simulink model "gm_uz_pmsm_model_9ph_vnl"  (R2021b)
settings: Solver=FixedStepAuto  StartTime=0.0  StopTime=0.8  RelTol=1e-3
PreLoadFcn:
  | uz_pmsm_model_9ph_init_parameter
undefined symbols (not defined in the file or in its folder): a, b, c, friction_coefficient, inertia, k_i_d, k_i_q, k_p_d, k_p_q, Kpd, L_d, L_o1, L_o2, L_q, L_x1, L_x2, L_y1, L_y2, L_zero, polepair, psi_pm, R_1, static_friction_torque, Tnd, ts
libraries: hdlmdlgenlib x191, hdlsllib x90, dspsigops x19, simulink x17, slpidlib x2, spsAlphaBetaZerotodq0Lib x1, pid_lib x1, spsdq0toAlphaBetaZeroLib x1
(part 1 of 7)
settings Model: Creator=ts  LastModifiedBy=valen
settings SolverCC: AlgebraicLoopSolver=TrustRegion  AutoInsertRateTranBlk=on
settings DataIOCC: LimitDataPoints=on  SaveOutput=off  SaveTime=off
settings OptimizationCC: BlockReduction=off  ConditionallyExecuteInputs=off  DefaultParameterBehavior=Inlined  LifeSpan=inf
settings DebuggingCC: AlgebraicLoopMsg=error  ArtificialAlgebraicLoopMsg=none  InheritedTsInSrcMsg=none  SingleTaskRateTransMsg=error  AllowSymbolicDim=off  StrictBusMsg=ErrorOnBusTreatedAsVector  SFUnexpectedBacktrackingDiag=warning  SFNoUnconditionalDefaultTransitionDiag=warning  SFExecutionAtInitializationDiag=none  SFMachineParentedDataDiag=warning  ArithmeticOperatorsInVariantConditions=warning
settings HardwareCC: ProdBitPerPointer=32  ProdBitPerSizeT=32  ProdBitPerPtrDiffT=32  ProdLargestAtomicFloat=None  ProdIntDivRoundTo=Undefined  ProdEndianess=Unspecified  ProdWordSize=32  ProdHWDeviceType=ASIC/FPGA->ASIC/FPGA  ProdEqTarget=off
settings SFSimCC: SimUseLocalCustomCode=off  CustomCodeUndefinedFunction=UseInterfaceOnly
settings RTWCC: RTWUseLocalCustomCode=off
settings CodeAppCC: StateflowObjectComments=on
settings GRTTargetCC: TargetLangStandard=C89/C90 (ANSI)
settings ConfigComp: CovScope=ReferencedModels  CovMetricSettings=dw  CovSaveCumulativeToWorkspaceVar=on  CovSaveSingleToWorkspaceVar=on  CovExternalEMLEnable=off  CovSFcnEnable=off

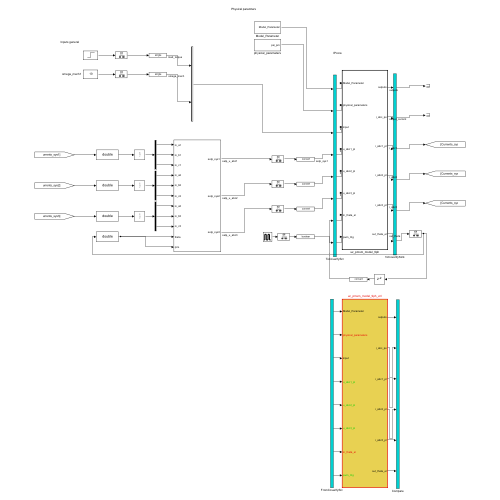
[thumbnail: Simulink's stored preview of the top-level diagram]
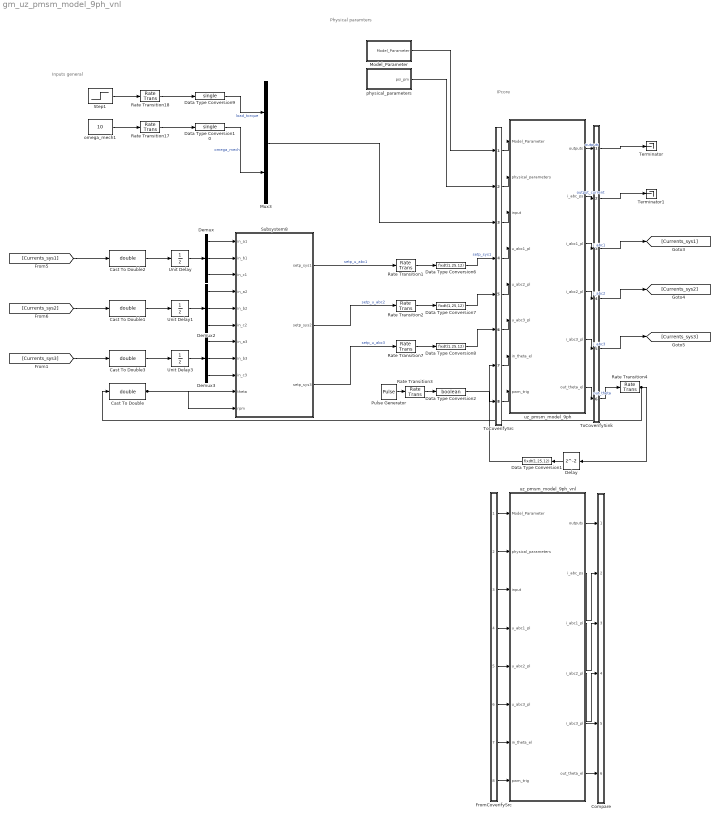
== system gm_uz_pmsm_model_9ph_vnl ==
  note: IPcore
  note: Physical paramters
  note: Inputs general
  Cast To Double{,1..3} (4 alike) : DataTypeConversion  OutDataTypeStr=double
  Compare : Subsystem
      mask Display: disp('')
  Data Type Conversion{1,6..8} (4 alike) : DataTypeConversion  OutDataTypeStr=fixdt(1,25,12)  RndMeth=Nearest
  Data Type Conversion10 : DataTypeConversion  OutDataTypeStr=single  RndMeth=Nearest
  Data Type Conversion2 : DataTypeConversion  OutDataTypeStr=boolean  RndMeth=Nearest
  Data Type Conversion9 : DataTypeConversion  OutDataTypeStr=single  RndMeth=Nearest
  Delay : Delay
  Demux : Demux  Outputs=3
  Demux2 : Demux  Outputs=3
  Demux3 : Demux  Outputs=3
  FromCoverifySrc : Subsystem
      mask Display: disp('')
  Model_Parameter : Subsystem
  Mux3 : Mux  Inputs=2
  Pulse Generator : DiscretePulseGenerator  PulseType=Time based  Period=1e-9  PulseWidth=50
  Rate Transition{1..4,7,17..18} (7 alike) : RateTransition  OutPortSampleTime=ts
  Step1 : Step  Time=0.25  After=20  SampleTime=0
  Subsystem8 : Subsystem
  Terminator : Terminator
  Terminator1 : Terminator
  ToCoverifySink : Subsystem
      mask Display: disp('')
  ToCoverifySrc : Subsystem
      mask Display: disp('')
  Unit Delay : UnitDelay  SampleTime=-1  HasFrameUpgradeWarning=on
  Unit Delay1 : UnitDelay  SampleTime=-1  HasFrameUpgradeWarning=on
  Unit Delay3 : UnitDelay  SampleTime=-1  HasFrameUpgradeWarning=on
  omega_mech1 : Constant  Value=10
  physical_parameters : Subsystem
  uz_pmsm_model_9ph : Subsystem  TreatAsAtomicUnit=on
  uz_pmsm_model_9ph_vnl : Subsystem  TreatAsAtomicUnit=on
  wires:
  omega_mech1/1 -> Rate Transition17/1
  Rate Transition18/1 -> Data Type Conversion9/1
  Step1/1 -> Rate Transition18/1
  Data Type Conversion10/1 -> Mux3/2  "omega_mech"
  Rate Transition17/1 -> Data Type Conversion10/1
  Data Type Conversion9/1 -> Mux3/1  "load_torque"
  Delay/1 -> Data Type Conversion1/1
  Subsystem8/1(setp_sys1) -> Rate Transition1/1  "setp_u_abc1"
  Subsystem8/2(setp_sys2) -> Rate Transition2/1  "setp_u_abc2"
  Subsystem8/3(setp_sys3) -> Rate Transition7/1  "setp_u_abc3"
  Unit Delay3/1 -> Demux3/1
  Demux/2 -> Subsystem8/2(in_b1)
  Demux2/1 -> Subsystem8/4(in_a2)
  Demux3/2 -> Subsystem8/8(in_b3)
  Unit Delay1/1 -> Demux2/1
  Demux/3 -> Subsystem8/3(in_c1)
  [Currents_sys1] -> Cast To Double2/1
  [Currents_sys2] -> Cast To Double1/1
  Demux3/3 -> Subsystem8/9(in_c3)
  Unit Delay/1 -> Demux/1
  [Currents_sys3] -> Cast To Double3/1
  Demux3/1 -> Subsystem8/7(in_a3)
  Demux/1 -> Subsystem8/1(in_a1)
  Demux2/2 -> Subsystem8/5(in_b2)
  Demux2/3 -> Subsystem8/6(in_c2)
  Cast To Double/1 -> Subsystem8/11(rpm), Subsystem8/10(theta)
  Cast To Double1/1 -> Unit Delay1/1
  Cast To Double2/1 -> Unit Delay/1
  Cast To Double3/1 -> Unit Delay3/1
  Rate Transition1/1 -> Data Type Conversion6/1
  Rate Transition2/1 -> Data Type Conversion7/1
  Rate Transition7/1 -> Data Type Conversion8/1
  Rate Transition3/1 -> Data Type Conversion2/1
  Pulse Generator/1 -> Rate Transition3/1
  Rate Transition4/1 -> Delay/1, Cast To Double/1
  ToCoverifySrc/1(out1) -> uz_pmsm_model_9ph/1(Model_Parameter)
  ToCoverifySrc/2(out2) -> uz_pmsm_model_9ph/2(physical_parameters)
  ToCoverifySrc/3(out3) -> uz_pmsm_model_9ph/3(input)
  ToCoverifySrc/4(out4) -> uz_pmsm_model_9ph/4(u_abc1_pl)
  ToCoverifySrc/5(out5) -> uz_pmsm_model_9ph/5(u_abc2_pl)
  ToCoverifySrc/6(out6) -> uz_pmsm_model_9ph/6(u_abc3_pl)
  ToCoverifySrc/7(out7) -> uz_pmsm_model_9ph/7(in_theta_el)
  ToCoverifySrc/8(out8) -> uz_pmsm_model_9ph/8(pwm_trig)
  uz_pmsm_model_9ph/1(outputs) -> ToCoverifySink/1(in1)  "outputs"
  uz_pmsm_model_9ph/2(i_abc_ps) -> ToCoverifySink/2(in2)  "output_current"
  uz_pmsm_model_9ph/3(i_abc1_pl) -> ToCoverifySink/3(in3)  "i_abc1"
  uz_pmsm_model_9ph/4(i_abc2_pl) -> ToCoverifySink/4(in4)  "i_abc2"
  uz_pmsm_model_9ph/5(i_abc3_pl) -> ToCoverifySink/5(in5)  "i_abc3"
  uz_pmsm_model_9ph/6(out_theta_el) -> ToCoverifySink/6(in6)  "out_theta"
  Model_Parameter/1(Model_Parameter) -> ToCoverifySrc/1(in1)
  physical_parameters/1(psi_pm) -> ToCoverifySrc/2(in2)
  Mux3/1 -> ToCoverifySrc/3(in3)
  Data Type Conversion6/1 -> ToCoverifySrc/4(in4)  "setp_sys1"
  Data Type Conversion7/1 -> ToCoverifySrc/5(in5)
  Data Type Conversion8/1 -> ToCoverifySrc/6(in6)
  Data Type Conversion1/1 -> ToCoverifySrc/7(in7)
  Data Type Conversion2/1 -> ToCoverifySrc/8(in8)
  ToCoverifySink/1(out1) -> Terminator/1
  ToCoverifySink/2(out2) -> Terminator1/1
  ToCoverifySink/3(out3) -> [Currents_sys1]
  ToCoverifySink/4(out4) -> [Currents_sys2]
  ToCoverifySink/5(out5) -> [Currents_sys3]
  ToCoverifySink/6(out6) -> Rate Transition4/1
  FromCoverifySrc/1(out1) -> uz_pmsm_model_9ph_vnl/1(Model_Parameter)
  FromCoverifySrc/2(out2) -> uz_pmsm_model_9ph_vnl/2(physical_parameters)
  FromCoverifySrc/3(out3) -> uz_pmsm_model_9ph_vnl/3(input)
  FromCoverifySrc/4(out4) -> uz_pmsm_model_9ph_vnl/4(u_abc1_pl)
  FromCoverifySrc/5(out5) -> uz_pmsm_model_9ph_vnl/5(u_abc2_pl)
  FromCoverifySrc/6(out6) -> uz_pmsm_model_9ph_vnl/6(u_abc3_pl)
  FromCoverifySrc/7(out7) -> uz_pmsm_model_9ph_vnl/7(in_theta_el)
  FromCoverifySrc/8(out8) -> uz_pmsm_model_9ph_vnl/8(pwm_trig)
  uz_pmsm_model_9ph_vnl/1(outputs) -> Compare/1(in1)
  uz_pmsm_model_9ph_vnl/2(i_abc_ps) -> Compare/2(in2)
  uz_pmsm_model_9ph_vnl/3(i_abc1_pl) -> Compare/3(in3)
  uz_pmsm_model_9ph_vnl/4(i_abc2_pl) -> Compare/4(in4)
  uz_pmsm_model_9ph_vnl/5(i_abc3_pl) -> Compare/5(in5)
  uz_pmsm_model_9ph_vnl/6(out_theta_el) -> Compare/6(in6)

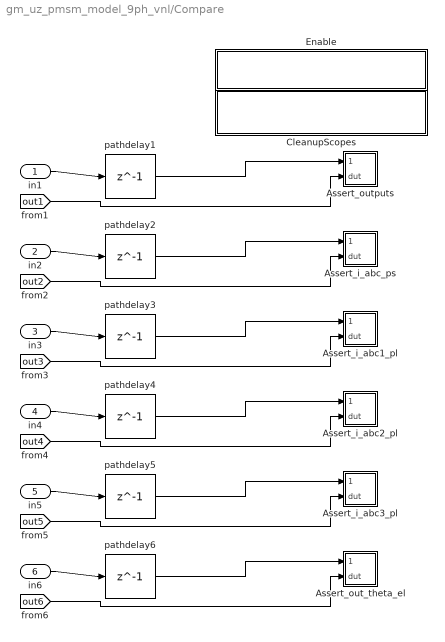
== system gm_uz_pmsm_model_9ph_vnl/Compare ==
  in1 : Inport
  in2 : Inport  Port=2
  in3 : Inport  Port=3
  in4 : Inport  Port=4
  in5 : Inport  Port=5
  in6 : Inport  Port=6
  Assert_i_abc1_pl : Subsystem
  Assert_i_abc2_pl : Subsystem
  Assert_i_abc3_pl : Subsystem
  Assert_i_abc_ps : Subsystem  mask{ToleranceValue=1e-07}
  Assert_out_theta_el : Subsystem
  Assert_outputs : Subsystem  mask{ToleranceValue=1e-07}
  CleanupScopes : Subsystem
      settings: OpenFcn=|
      | blkName = gcb; %self block
      | idx = regexp(blkName, '/CleanupScopes$', 'once');
      | blkParent = blkName(1:idx-1);
      | blks=find_system(blkParent, 'LookUnderMasks', 'all','blocktype', 'Scope');
      | for itr = 1:length(blks)
      | 	 hScopeCfg = get_param(blks{itr},'ScopeConfiguration');
      | 	 hScopeCfg.Visible = ~ hScopeCfg.Visible;
      | end
      | drawnow;
      mask Display: fprintf(message('hdlcoder:cosim:vnl_dblclick').getString());
  Enable : Subsystem
      settings: OpenFcn=|
      | blkName = gcb;
      | idx = regexp(blkName, '/Enable$', 'once');
      | blkParent = blkName(1:idx-1);
      | blks=find_system(blkParent, 'LookUnderMasks', 'all','blocktype', 'Assertion');
      | e = get_param(blks{1}, 'Enabled');
      | if strcmp(e, 'on'), f= 'off';, else, f = 'on';, end
      | for ii=1:length(blks), set_param(blks{ii}, 'Enabled', f);, end
      | set_param(gcb, 'MaskDisplay',['fprintf(message(''hdlcoder:cosim:vnl_dblclick_assertions'',','''',upper(e),'''',').getString())']);
      mask Display: fprintf(message('hdlcoder:cosim:vnl_dblclick_assertions','OFF').getString());
  pathdelay{1..6} (6 alike) : Delay  DelayLength=1
  wires:
  in1/1 -> pathdelay1/1
  pathdelay1/1 -> Assert_outputs/1(cosim)
  [out1] -> Assert_outputs/2(dut)
  in2/1 -> pathdelay2/1
  pathdelay2/1 -> Assert_i_abc_ps/1(cosim)
  [out2] -> Assert_i_abc_ps/2(dut)
  in3/1 -> pathdelay3/1
  pathdelay3/1 -> Assert_i_abc1_pl/1(cosim)
  [out3] -> Assert_i_abc1_pl/2(dut)
  in4/1 -> pathdelay4/1
  pathdelay4/1 -> Assert_i_abc2_pl/1(cosim)
  [out4] -> Assert_i_abc2_pl/2(dut)
  in5/1 -> pathdelay5/1
  pathdelay5/1 -> Assert_i_abc3_pl/1(cosim)
  [out5] -> Assert_i_abc3_pl/2(dut)
  in6/1 -> pathdelay6/1
  pathdelay6/1 -> Assert_out_theta_el/1(cosim)
  [out6] -> Assert_out_theta_el/2(dut)

== system gm_uz_pmsm_model_9ph_vnl/FromCoverifySrc ==
  out1 : Outport
  out2 : Outport  Port=2
  out3 : Outport  Port=3
  out4 : Outport  Port=4
  out5 : Outport  Port=5
  out6 : Outport  Port=6
  out7 : Outport  Port=7
  out8 : Outport  Port=8
  wires:
  [in1] -> out1/1
  [in2] -> out2/1
  [in3] -> out3/1
  [in4] -> out4/1
  [in5] -> out5/1
  [in6] -> out6/1
  [in7] -> out7/1
  [in8] -> out8/1

== system gm_uz_pmsm_model_9ph_vnl/Model_Parameter ==
  note: This flag determines if omega_mech is used as an input value or
      | if the mechanical system is simulated by the model
  Bus Creator : BusCreator  Inputs=4
  Constant3 : Constant  Value=0
  Data Type Conversion{3..4,9..10} (4 alike) : DataTypeConversion  OutDataTypeStr=boolean
  Rate Transition{6,8,17..18} (4 alike) : RateTransition  OutPortSampleTime=ts
  simulate_mechanical : Constant  Value=false
  simulate_mechanical1 : Constant  Value=false
  simulate_mechanical2 : Constant  Value=false
  Model_Parameter : Outport
  wires:
  simulate_mechanical2/1 -> Rate Transition18/1
  simulate_mechanical/1 -> Rate Transition8/1
  Rate Transition8/1 -> Data Type Conversion4/1
  Rate Transition6/1 -> Data Type Conversion3/1
  Constant3/1 -> Rate Transition6/1
  simulate_mechanical1/1 -> Rate Transition17/1
  Rate Transition17/1 -> Data Type Conversion9/1
  Rate Transition18/1 -> Data Type Conversion10/1
  Data Type Conversion10/1 -> Bus Creator/4  "control_dq_abc"
  Data Type Conversion9/1 -> Bus Creator/3  "switch_pspl"
  Data Type Conversion4/1 -> Bus Creator/2  "simulate_mechanical"
  Bus Creator/1 -> Model_Parameter/1
  Data Type Conversion3/1 -> Bus Creator/1  "reset_integrators"

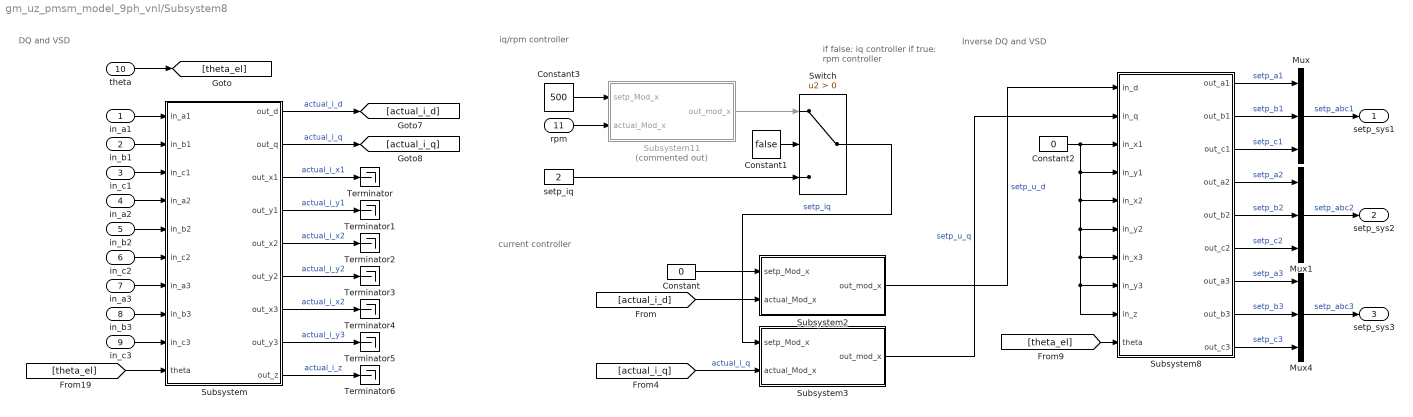
== system gm_uz_pmsm_model_9ph_vnl/Subsystem8 ==
  note: DQ and VSD
  note: current controller
  note: iq/rpm controller
  note: if false: iq controller
      | if true: rpm controller
  note: Inverse DQ and VSD
  in_a1 : Inport
  in_b1 : Inport  Port=2
  in_c1 : Inport  Port=3
  in_a2 : Inport  Port=4
  in_b2 : Inport  Port=5
  in_c2 : Inport  Port=6
  in_a3 : Inport  Port=7
  in_b3 : Inport  Port=8
  in_c3 : Inport  Port=9
  theta : Inport  Port=10
  rpm : Inport  Port=11
  Constant : Constant  Value=0
  Constant1 : Constant  Value=false
  Constant2 : Constant  Value=0
  Constant3 : Constant  Value=500
  Mux : Mux  Inputs=3
  Mux1 : Mux  Inputs=3
  Mux4 : Mux  Inputs=3
  Subsystem : Subsystem
  Subsystem11 : Subsystem  Commented=on
  Subsystem2 : Subsystem
  Subsystem3 : Subsystem
  Subsystem8 : Subsystem
  Switch : Switch  Criteria=u2 > Threshold
  Terminator{,1..6} (7 alike) : Terminator
  setp_iq : Constant  Value=2
  setp_sys1 : Outport
  setp_sys2 : Outport  Port=2
  setp_sys3 : Outport  Port=3
  wires:
  Subsystem/4(out_y1) -> Terminator1/1  "actual_i_y1"
  Subsystem8/1(out_a1) -> Mux/1  "setp_a1"
  in_b1/1 -> Subsystem/2(in_b1)
  [theta_el] -> Subsystem8/10(theta)
  Subsystem8/2(out_b1) -> Mux/2  "setp_b1"
  Subsystem8/3(out_c1) -> Mux/3  "setp_c1"
  Subsystem/3(out_x1) -> Terminator/1  "actual_i_x1"
  in_c1/1 -> Subsystem/3(in_c1)
  [actual_i_d] -> Subsystem2/2(actual_Mod_x)
  Constant/1 -> Subsystem2/1(setp_Mod_x)
  Subsystem/6(out_y2) -> Terminator3/1  "actual_i_y2"
  Subsystem/5(out_x2) -> Terminator2/1  "actual_i_x2"
  in_a1/1 -> Subsystem/1(in_a1)
  [actual_i_q] -> Subsystem3/2(actual_Mod_x)  "actual_i_q"
  in_b2/1 -> Subsystem/5(in_b2)
  in_a2/1 -> Subsystem/4(in_a2)
  in_c2/1 -> Subsystem/6(in_c2)
  theta/1 -> [theta_el]
  Mux/1 -> setp_sys1/1  "setp_abc1"
  Subsystem/8(out_y3) -> Terminator5/1  "actual_i_y3"
  Subsystem/7(out_x3) -> Terminator4/1  "actual_i_x2"
  Subsystem/9(out_z) -> Terminator6/1  "actual_i_z"
  in_c3/1 -> Subsystem/9(in_c3)
  in_b3/1 -> Subsystem/8(in_b3)
  in_a3/1 -> Subsystem/7(in_a3)
  Mux1/1 -> setp_sys2/1  "setp_abc2"
  Subsystem8/6(out_c2) -> Mux1/3  "setp_c2"
  Subsystem8/5(out_b2) -> Mux1/2  "setp_b2"
  Subsystem8/4(out_a2) -> Mux1/1  "setp_a2"
  Mux4/1 -> setp_sys3/1  "setp_abc3"
  Subsystem8/7(out_a3) -> Mux4/1  "setp_a3"
  Subsystem8/8(out_b3) -> Mux4/2  "setp_b3"
  Subsystem8/9(out_c3) -> Mux4/3  "setp_c3"
  rpm/1 -> Subsystem11/2(actual_Mod_x)
  Subsystem/1(out_d) -> [actual_i_d]  "actual_i_d"
  Subsystem/2(out_q) -> [actual_i_q]  "actual_i_q"
  [theta_el] -> Subsystem/10(theta)
  Constant2/1 -> Subsystem8/3(in_x1), Subsystem8/8(in_y3), Subsystem8/9(in_z), Subsystem8/7(in_x3), Subsystem8/6(in_y2), Subsystem8/5(in_x2), Subsystem8/4(in_y1)
  Subsystem11/1(out_mod_x) -> Switch/1
  Switch/1 -> Subsystem3/1(setp_Mod_x)  "setp_iq"
  Constant1/1 -> Switch/2
  setp_iq/1 -> Switch/3
  Constant3/1 -> Subsystem11/1(setp_Mod_x)
  Subsystem3/1(out_mod_x) -> Subsystem8/2(in_q)  "setp_u_q"
  Subsystem2/1(out_mod_x) -> Subsystem8/1(in_d)  "setp_u_d"

== system gm_uz_pmsm_model_9ph_vnl/ToCoverifySink ==
  in1 : Inport
  in2 : Inport  Port=2
  in3 : Inport  Port=3
  in4 : Inport  Port=4
  in5 : Inport  Port=5
  in6 : Inport  Port=6
  out1 : Outport
  out2 : Outport  Port=2
  out3 : Outport  Port=3
  out4 : Outport  Port=4
  out5 : Outport  Port=5
  out6 : Outport  Port=6
  tag scope: out1=global, out2=global, out3=global, out4=global, out5=global, out6=global
  wires:
  in1/1 -> out1/1, [out1]
  in2/1 -> out2/1, [out2]
  in3/1 -> out3/1, [out3]
  in4/1 -> out4/1, [out4]
  in5/1 -> out5/1, [out5]
  in6/1 -> out6/1, [out6]

== system gm_uz_pmsm_model_9ph_vnl/ToCoverifySrc ==
  in1 : Inport
  in2 : Inport  Port=2
  in3 : Inport  Port=3
  in4 : Inport  Port=4
  in5 : Inport  Port=5
  in6 : Inport  Port=6
  in7 : Inport  Port=7
  in8 : Inport  Port=8
  out1 : Outport
  out2 : Outport  Port=2
  out3 : Outport  Port=3
  out4 : Outport  Port=4
  out5 : Outport  Port=5
  out6 : Outport  Port=6
  out7 : Outport  Port=7
  out8 : Outport  Port=8
  tag scope: in1=global, in2=global, in3=global, in4=global, in5=global, in6=global, in7=global, in8=global
  wires:
  in1/1 -> out1/1, [in1]
  in2/1 -> out2/1, [in2]
  in3/1 -> out3/1, [in3]
  in4/1 -> out4/1, [in4]
  in5/1 -> out5/1, [in5]
  in6/1 -> out6/1, [in6]
  in7/1 -> out7/1, [in7]
  in8/1 -> out8/1, [in8]

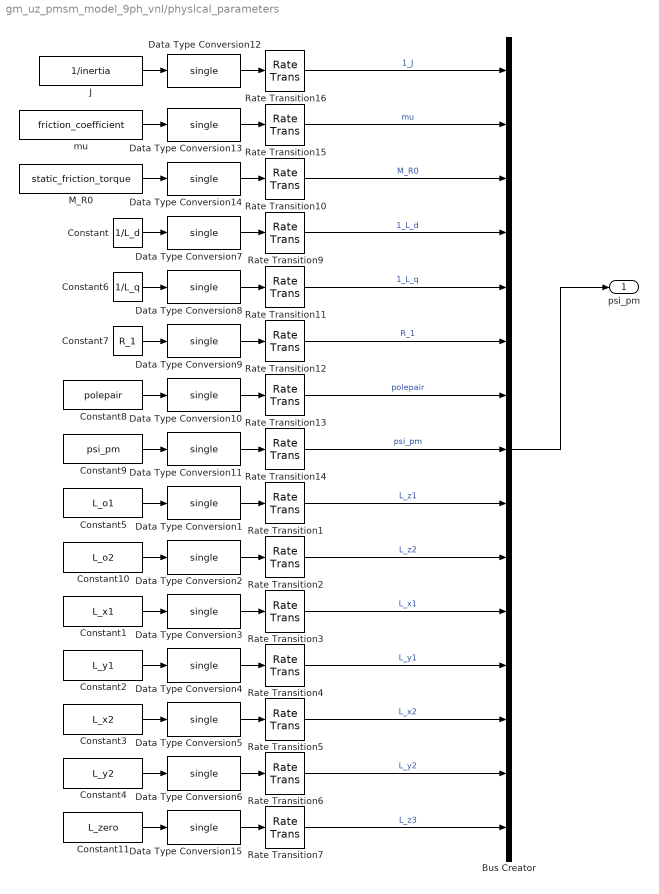
== system gm_uz_pmsm_model_9ph_vnl/physical_parameters ==
  Bus Creator : BusCreator  Inputs=15
  Constant : Constant  Value=1/L_d
  Constant1 : Constant  Value=L_x1
  Constant10 : Constant  Value=L_o2
  Constant11 : Constant  Value=L_zero
  Constant2 : Constant  Value=L_y1
  Constant3 : Constant  Value=L_x2
  Constant4 : Constant  Value=L_y2
  Constant5 : Constant  Value=L_o1
  Constant6 : Constant  Value=1/L_q
  Constant7 : Constant  Value=R_1
  Constant8 : Constant  Value=polepair
  Constant9 : Constant  Value=psi_pm
  Data Type Conversion{1..15} (15 alike) : DataTypeConversion  OutDataTypeStr=single
  J : Constant  Value=1/inertia
  M_R0 : Constant  Value=static_friction_torque
  Rate Transition{1..7,9..16} (15 alike) : RateTransition  OutPortSampleTime=ts
  mu : Constant  Value=friction_coefficient
  psi_pm : Outport
  wires:
  Data Type Conversion12/1 -> Rate Transition16/1
  Data Type Conversion7/1 -> Rate Transition9/1
  Rate Transition10/1 -> Bus Creator/3  "M_R0"
  Rate Transition14/1 -> Bus Creator/8  "psi_pm"
  Data Type Conversion14/1 -> Rate Transition10/1
  Rate Transition12/1 -> Bus Creator/6  "R_1"
  Rate Transition16/1 -> Bus Creator/1  "1_J"
  Rate Transition13/1 -> Bus Creator/7  "polepair"
  Bus Creator/1 -> psi_pm/1
  Data Type Conversion11/1 -> Rate Transition14/1
  Constant8/1 -> Data Type Conversion10/1
  Data Type Conversion9/1 -> Rate Transition12/1
  Rate Transition15/1 -> Bus Creator/2  "mu"
  Constant6/1 -> Data Type Conversion8/1
  Rate Transition9/1 -> Bus Creator/4  "1_L_d"
  J/1 -> Data Type Conversion12/1
  Data Type Conversion8/1 -> Rate Transition11/1
  Data Type Conversion10/1 -> Rate Transition13/1
  mu/1 -> Data Type Conversion13/1
  M_R0/1 -> Data Type Conversion14/1
  Rate Transition11/1 -> Bus Creator/5  "1_L_q"
  Data Type Conversion13/1 -> Rate Transition15/1
  Constant7/1 -> Data Type Conversion9/1
  Constant9/1 -> Data Type Conversion11/1
  Constant/1 -> Data Type Conversion7/1
  Data Type Conversion1/1 -> Rate Transition1/1
  Data Type Conversion2/1 -> Rate Transition2/1
  Data Type Conversion3/1 -> Rate Transition3/1
  Data Type Conversion4/1 -> Rate Transition4/1
  Data Type Conversion5/1 -> Rate Transition5/1
  Data Type Conversion6/1 -> Rate Transition6/1
  Constant11/1 -> Data Type Conversion15/1
  Data Type Conversion15/1 -> Rate Transition7/1
  Rate Transition1/1 -> Bus Creator/9  "L_z1"
  Rate Transition7/1 -> Bus Creator/15  "L_z3"
  Rate Transition6/1 -> Bus Creator/14  "L_y2"
  Rate Transition5/1 -> Bus Creator/13  "L_x2"
  Rate Transition4/1 -> Bus Creator/12  "L_y1"
  Rate Transition3/1 -> Bus Creator/11  "L_x1"
  Rate Transition2/1 -> Bus Creator/10  "L_z2"
  Constant4/1 -> Data Type Conversion6/1
  Constant3/1 -> Data Type Conversion5/1
  Constant2/1 -> Data Type Conversion4/1
  Constant1/1 -> Data Type Conversion3/1
  Constant5/1 -> Data Type Conversion1/1
  Constant10/1 -> Data Type Conversion2/1
